simulink model "imc_Q_c"  (Simulink 5.0)
settings: Solver=ode45  StartTime=t0  StopTime=tf  RelTol=1e-3
values from neighbouring files (symbols this model uses):
  A = [1 -0.44]    [visc_imc.m]
  alpha = 0.5    [vande_imc.m]    (also in vande_imc_general.m; visc_imc.m)
  B = [0.51 1.21]    [visc_imc.m]
  den = [1 4.6429 5.3821]    [vande_imc.m]    (also in vande_imc_general.m)
  num = [-1.117 3.1472]    [vande_imc.m]    (also in vande_imc_general.m)
  Ts = 0.1    [vande_imc.m]    (also in vande_imc_general.m)
undefined symbols (not defined in the file or in its folder): GiD, GiN, Nvar, st, tau, zk
settings Model: Creator=kannanm  LastModifiedBy=kannan  ExtModeAutoUpdateStatusClock=off

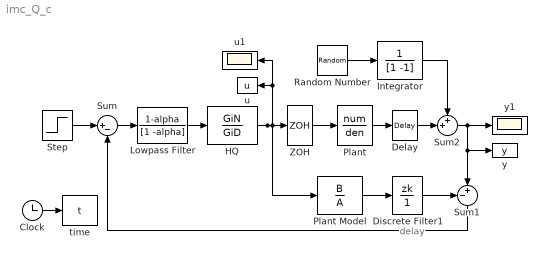
== system imc_Q_c ==
  note: delay
  Clock : Clock
      settings: Decimation=10
  Delay : TransportDelay  DelayTime=tau
  Discrete Filter1 : DiscreteFilter  Numerator=zk  Denominator=1  SampleTime=Ts
  HQ : DiscreteFilter  Numerator=GiN  Denominator=GiD  SampleTime=Ts
  Integrator : DiscreteFilter  Numerator=1  Denominator=[1 -1]  SampleTime=Ts
  Lowpass Filter : DiscreteFilter  Numerator=1-alpha  Denominator=[1 -alpha]  SampleTime=Ts
  Plant : TransferFcn  Numerator=num  Denominator=den
  Plant Model : DiscreteFilter  Numerator=B  Denominator=A  SampleTime=Ts
  Random Number : RandomNumber  Variance=Nvar  SampleTime=Ts
  Step : Step  After=st  SampleTime=Ts
  Sum : Sum  Inputs=|+-  SaturateOnIntegerOverflow=on
  Sum1 : Sum  Orientation=down  Inputs=-+|  SaturateOnIntegerOverflow=on
  Sum2 : Sum  Inputs=++|  SaturateOnIntegerOverflow=on
  ZOH : ZeroOrderHold  SampleTime=Ts
  time : ToWorkspace  VariableName=t  SampleTime=Ts  SaveFormat=Array
  u : ToWorkspace  VariableName=u  SampleTime=Ts  SaveFormat=Array
  u1 : Scope
  y : ToWorkspace  VariableName=y  SampleTime=Ts  SaveFormat=Array
  y1 : Scope
  wires:
  Lowpass Filter/1 -> HQ/1
  HQ/1 -> Plant Model/1, ZOH/1, u1/1, u/1
  Sum/1 -> Lowpass Filter/1
  Plant Model/1 -> Discrete Filter1/1
  Plant/1 -> Delay/1
  Sum1/1 -> Sum/2
  Step/1 -> Sum/1
  Integrator/1 -> Sum2/1
  Sum2/1 -> y1/1, Sum1/2, y/1
  Discrete Filter1/1 -> Sum1/1
  Random Number/1 -> Integrator/1
  Clock/1 -> time/1
  ZOH/1 -> Plant/1
  Delay/1 -> Sum2/2
